simulink model "Control"  (R2022a)
settings: Solver=VariableStepAuto  StartTime=0.0  StopTime=10.0  RelTol=1e-3
libraries: slpidlib x6, robotcorelib x1
settings Model: LastModifiedBy=s389152

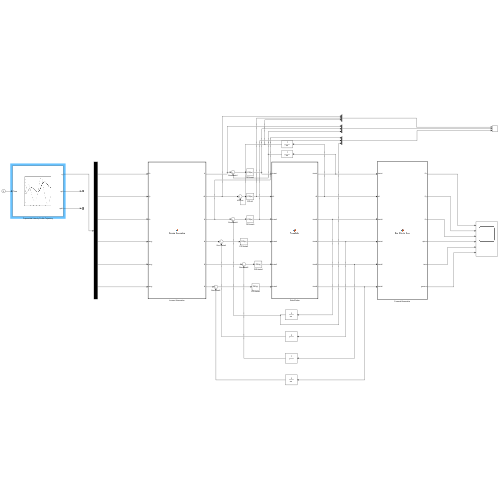
[thumbnail: Simulink's stored preview of the top-level diagram]
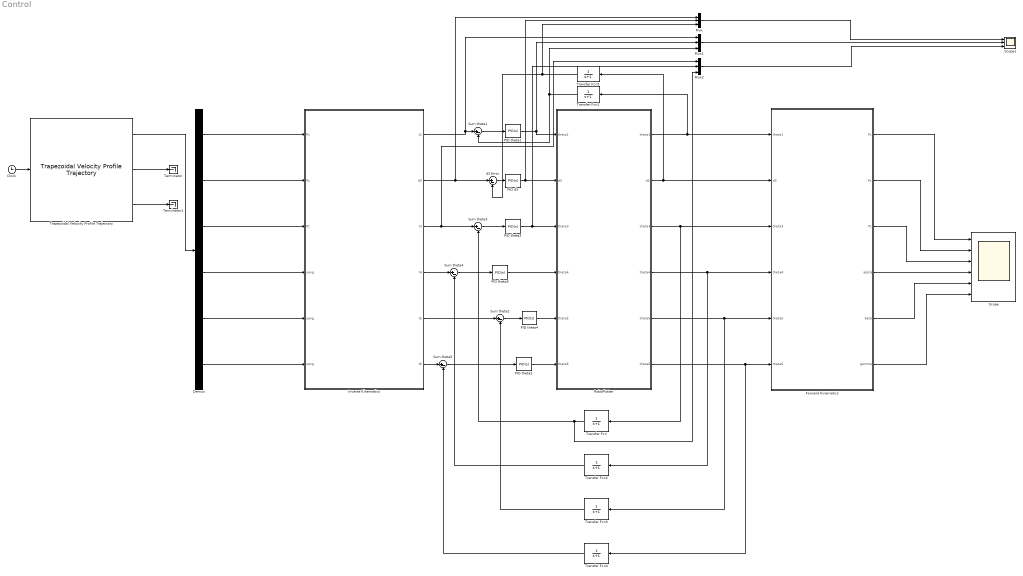
== system Control ==
  Clock : Clock
      settings: Decimation=5
  Demux : Demux  Outputs=6
  Forward Kinematics : MATLAB Function  TreatAsAtomicUnit=on
  Inverse Kinematics : MATLAB Function  TreatAsAtomicUnit=on
  Mux : Mux  Inputs=3
  Mux1 : Mux  Inputs=3
  Mux2 : Mux  Inputs=3
  PID d3 : slpidlib/PID Controller  Controller=PID  Form=Parallel  TimeDomain=Continuous-time  UseExternalTs=off  SampleTime=-1  IntegratorMethod=Forward Euler  FilterMethod=Forward Euler  ControllerParametersSource=internal  P=2  I=1.3  UseKiTs=off  D=.01  N=100  UseFilter=on  TunerSelectOption=Transfer Function Based (PID Tuner App)  InitialConditionSource=internal  InitialConditionForIntegrator=0  InitialConditionForFilter=0  DifferentiatorICPrevScaledInput=0  ExternalReset=none  TrackingMode=off  Kt=1  LimitOutput=off  SatLimitsSource=internal  UpperSaturationLimit=inf  LowerSaturationLimit=-inf  LinearizeAsGain=on  AntiWindupMode=none  Kb=1  POutMin=[]  POutMax=[]  IOutMin=[]  IOutMax=[]  DOutMin=[]  DOutMax=[]  NOutMin=[]  NOutMax=[]  SumOutMin=[]  SumOutMax=[]  SaturationOutMin=[]  SaturationOutMax=[]  PParamMin=[]  PParamMax=[]  IParamMin=[]  IParamMax=[]  DParamMin=[]  DParamMax=[]  NParamMin=[]  NParamMax=[]  KbParamMin=[]  KbParamMax=[]  KtParamMin=[]  KtParamMax=[]  KbOutMin=[]  KbOutMax=[]  KtOutMin=[]  KtOutMax=[]  IntegratorOutMin=[]  IntegratorOutMax=[]  FilterOutMin=[]  FilterOutMax=[]  SumI1OutMin=[]  SumI1OutMax=[]  SumI2OutMin=[]  SumI2OutMax=[]  SumI3OutMin=[]  SumI3OutMax=[]  SumI4OutMin=[]  SumI4OutMax=[]  SumDOutMin=[]  SumDOutMax=[]  DifferentiatorOutMin=[]  DifferentiatorOutMax=[]  FilterDiffOutCoefMin=[]  FilterDiffOutCoefMax=[]  ReciprocalOutMin=[]  ReciprocalOutMax=[]  SumDenOutMin=[]  SumDenOutMax=[]  SumNumOutMin=[]  SumNumOutMax=[]  DivideOutMin=[]  DivideOutMax=[]  UdiffTsProdOutMin=[]  UdiffTsProdOutMax=[]  NTsProdOutMin=[]  NTsProdOutMax=[]  UintegralTsProdOutMin=[]  UintegralTsProdOutMax=[]  UngainTsProdOutMin=[]  UngainTsProdOutMax=[]  IntegratorContinuousStateAttributes=''  IntegratorStateMustResolveToSignalObject=off  IntegratorRTWStateStorageClass=Auto  FilterContinuousStateAttributes=''  FilterStateMustResolveToSignalObject=off  FilterRTWStateStorageClass=Auto  ParallelPVariant=InternalParameters  IdealPVariant=Disabled  IVariant=InternalParameters  DVariant=InternalParameters  IntegratorVariant=Continuous  SatVariant=Disabled  AWVariant=Passthrough  PCopyVariant=Disabled  TRVariant=Disabled  FdbkBlocksVariant=Forward  IdealPFdbkVariant=Disabled  SatFdbkVariant=Disabled  DerivativeFilterVariant=ContFilter  NVariant=InternalParameters  NCopyVariant=Disabled  FilterICVariant=InternalICsFilter  IntegratorICVariant=InternalICs  ExternalResetVariant=Disabled  TRSumVariant=Passthrough  SumFdbkVariant=Disabled  SumVariant=Sum_PID  TsampFilterVariant=InternalTs  TsampNgainVariant=Passthrough  TsampIntegralVariant=Passthrough  ExternalSaturationOutDataTypeStr=Inherit: Same as second input  aMode=0
  PID theta1 : slpidlib/PID Controller  Controller=PID  Form=Parallel  TimeDomain=Continuous-time  UseExternalTs=off  SampleTime=-1  IntegratorMethod=Forward Euler  FilterMethod=Forward Euler  ControllerParametersSource=internal  P=1.3  I=1.3  UseKiTs=off  D=0.01  N=100  UseFilter=on  TunerSelectOption=Transfer Function Based (PID Tuner App)  InitialConditionSource=internal  InitialConditionForIntegrator=0  InitialConditionForFilter=0  DifferentiatorICPrevScaledInput=0  ExternalReset=none  TrackingMode=off  Kt=1  LimitOutput=off  SatLimitsSource=internal  UpperSaturationLimit=inf  LowerSaturationLimit=-inf  LinearizeAsGain=on  AntiWindupMode=none  Kb=1  POutMin=[]  POutMax=[]  IOutMin=[]  IOutMax=[]  DOutMin=[]  DOutMax=[]  NOutMin=[]  NOutMax=[]  SumOutMin=[]  SumOutMax=[]  SaturationOutMin=[]  SaturationOutMax=[]  PParamMin=[]  PParamMax=[]  IParamMin=[]  IParamMax=[]  DParamMin=[]  DParamMax=[]  NParamMin=[]  NParamMax=[]  KbParamMin=[]  KbParamMax=[]  KtParamMin=[]  KtParamMax=[]  KbOutMin=[]  KbOutMax=[]  KtOutMin=[]  KtOutMax=[]  IntegratorOutMin=[]  IntegratorOutMax=[]  FilterOutMin=[]  FilterOutMax=[]  SumI1OutMin=[]  SumI1OutMax=[]  SumI2OutMin=[]  SumI2OutMax=[]  SumI3OutMin=[]  SumI3OutMax=[]  SumI4OutMin=[]  SumI4OutMax=[]  SumDOutMin=[]  SumDOutMax=[]  DifferentiatorOutMin=[]  DifferentiatorOutMax=[]  FilterDiffOutCoefMin=[]  FilterDiffOutCoefMax=[]  ReciprocalOutMin=[]  ReciprocalOutMax=[]  SumDenOutMin=[]  SumDenOutMax=[]  SumNumOutMin=[]  SumNumOutMax=[]  DivideOutMin=[]  DivideOutMax=[]  UdiffTsProdOutMin=[]  UdiffTsProdOutMax=[]  NTsProdOutMin=[]  NTsProdOutMax=[]  UintegralTsProdOutMin=[]  UintegralTsProdOutMax=[]  UngainTsProdOutMin=[]  UngainTsProdOutMax=[]  IntegratorContinuousStateAttributes=''  IntegratorStateMustResolveToSignalObject=off  IntegratorRTWStateStorageClass=Auto  FilterContinuousStateAttributes=''  FilterStateMustResolveToSignalObject=off  FilterRTWStateStorageClass=Auto  ParallelPVariant=InternalParameters  IdealPVariant=Disabled  IVariant=InternalParameters  DVariant=InternalParameters  IntegratorVariant=Continuous  SatVariant=Disabled  AWVariant=Passthrough  PCopyVariant=Disabled  TRVariant=Disabled  FdbkBlocksVariant=Forward  IdealPFdbkVariant=Disabled  SatFdbkVariant=Disabled  DerivativeFilterVariant=ContFilter  NVariant=InternalParameters  NCopyVariant=Disabled  FilterICVariant=InternalICsFilter  IntegratorICVariant=InternalICs  ExternalResetVariant=Disabled  TRSumVariant=Passthrough  SumFdbkVariant=Disabled  SumVariant=Sum_PID  TsampFilterVariant=InternalTs  TsampNgainVariant=Passthrough  TsampIntegralVariant=Passthrough  ExternalSaturationOutDataTypeStr=Inherit: Same as second input  aMode=0
  PID theta2 : slpidlib/PID Controller  Controller=PID  Form=Parallel  TimeDomain=Continuous-time  UseExternalTs=off  SampleTime=-1  IntegratorMethod=Forward Euler  FilterMethod=Forward Euler  ControllerParametersSource=internal  P=1  I=1  UseKiTs=off  D=0  N=100  UseFilter=on  TunerSelectOption=Transfer Function Based (PID Tuner App)  InitialConditionSource=internal  InitialConditionForIntegrator=0  InitialConditionForFilter=0  DifferentiatorICPrevScaledInput=0  ExternalReset=none  TrackingMode=off  Kt=1  LimitOutput=off  SatLimitsSource=internal  UpperSaturationLimit=inf  LowerSaturationLimit=-inf  LinearizeAsGain=on  AntiWindupMode=none  Kb=1  POutMin=[]  POutMax=[]  IOutMin=[]  IOutMax=[]  DOutMin=[]  DOutMax=[]  NOutMin=[]  NOutMax=[]  SumOutMin=[]  SumOutMax=[]  SaturationOutMin=[]  SaturationOutMax=[]  PParamMin=[]  PParamMax=[]  IParamMin=[]  IParamMax=[]  DParamMin=[]  DParamMax=[]  NParamMin=[]  NParamMax=[]  KbParamMin=[]  KbParamMax=[]  KtParamMin=[]  KtParamMax=[]  KbOutMin=[]  KbOutMax=[]  KtOutMin=[]  KtOutMax=[]  IntegratorOutMin=[]  IntegratorOutMax=[]  FilterOutMin=[]  FilterOutMax=[]  SumI1OutMin=[]  SumI1OutMax=[]  SumI2OutMin=[]  SumI2OutMax=[]  SumI3OutMin=[]  SumI3OutMax=[]  SumI4OutMin=[]  SumI4OutMax=[]  SumDOutMin=[]  SumDOutMax=[]  DifferentiatorOutMin=[]  DifferentiatorOutMax=[]  FilterDiffOutCoefMin=[]  FilterDiffOutCoefMax=[]  ReciprocalOutMin=[]  ReciprocalOutMax=[]  SumDenOutMin=[]  SumDenOutMax=[]  SumNumOutMin=[]  SumNumOutMax=[]  DivideOutMin=[]  DivideOutMax=[]  UdiffTsProdOutMin=[]  UdiffTsProdOutMax=[]  NTsProdOutMin=[]  NTsProdOutMax=[]  UintegralTsProdOutMin=[]  UintegralTsProdOutMax=[]  UngainTsProdOutMin=[]  UngainTsProdOutMax=[]  IntegratorContinuousStateAttributes=''  IntegratorStateMustResolveToSignalObject=off  IntegratorRTWStateStorageClass=Auto  FilterContinuousStateAttributes=''  FilterStateMustResolveToSignalObject=off  FilterRTWStateStorageClass=Auto  ParallelPVariant=InternalParameters  IdealPVariant=Disabled  IVariant=InternalParameters  DVariant=InternalParameters  IntegratorVariant=Continuous  SatVariant=Disabled  AWVariant=Passthrough  PCopyVariant=Disabled  TRVariant=Disabled  FdbkBlocksVariant=Forward  IdealPFdbkVariant=Disabled  SatFdbkVariant=Disabled  DerivativeFilterVariant=ContFilter  NVariant=InternalParameters  NCopyVariant=Disabled  FilterICVariant=InternalICsFilter  IntegratorICVariant=InternalICs  ExternalResetVariant=Disabled  TRSumVariant=Passthrough  SumFdbkVariant=Disabled  SumVariant=Sum_PID  TsampFilterVariant=InternalTs  TsampNgainVariant=Passthrough  TsampIntegralVariant=Passthrough  ExternalSaturationOutDataTypeStr=Inherit: Same as second input  aMode=0
  PID theta3 : slpidlib/PID Controller  Controller=PID  Form=Parallel  TimeDomain=Continuous-time  UseExternalTs=off  SampleTime=-1  IntegratorMethod=Forward Euler  FilterMethod=Forward Euler  ControllerParametersSource=internal  P=1.3  I=1.3  UseKiTs=off  D=.01  N=100  UseFilter=on  TunerSelectOption=Transfer Function Based (PID Tuner App)  InitialConditionSource=internal  InitialConditionForIntegrator=0  InitialConditionForFilter=0  DifferentiatorICPrevScaledInput=0  ExternalReset=none  TrackingMode=off  Kt=1  LimitOutput=off  SatLimitsSource=internal  UpperSaturationLimit=inf  LowerSaturationLimit=-inf  LinearizeAsGain=on  AntiWindupMode=none  Kb=1  POutMin=[]  POutMax=[]  IOutMin=[]  IOutMax=[]  DOutMin=[]  DOutMax=[]  NOutMin=[]  NOutMax=[]  SumOutMin=[]  SumOutMax=[]  SaturationOutMin=[]  SaturationOutMax=[]  PParamMin=[]  PParamMax=[]  IParamMin=[]  IParamMax=[]  DParamMin=[]  DParamMax=[]  NParamMin=[]  NParamMax=[]  KbParamMin=[]  KbParamMax=[]  KtParamMin=[]  KtParamMax=[]  KbOutMin=[]  KbOutMax=[]  KtOutMin=[]  KtOutMax=[]  IntegratorOutMin=[]  IntegratorOutMax=[]  FilterOutMin=[]  FilterOutMax=[]  SumI1OutMin=[]  SumI1OutMax=[]  SumI2OutMin=[]  SumI2OutMax=[]  SumI3OutMin=[]  SumI3OutMax=[]  SumI4OutMin=[]  SumI4OutMax=[]  SumDOutMin=[]  SumDOutMax=[]  DifferentiatorOutMin=[]  DifferentiatorOutMax=[]  FilterDiffOutCoefMin=[]  FilterDiffOutCoefMax=[]  ReciprocalOutMin=[]  ReciprocalOutMax=[]  SumDenOutMin=[]  SumDenOutMax=[]  SumNumOutMin=[]  SumNumOutMax=[]  DivideOutMin=[]  DivideOutMax=[]  UdiffTsProdOutMin=[]  UdiffTsProdOutMax=[]  NTsProdOutMin=[]  NTsProdOutMax=[]  UintegralTsProdOutMin=[]  UintegralTsProdOutMax=[]  UngainTsProdOutMin=[]  UngainTsProdOutMax=[]  IntegratorContinuousStateAttributes=''  IntegratorStateMustResolveToSignalObject=off  IntegratorRTWStateStorageClass=Auto  FilterContinuousStateAttributes=''  FilterStateMustResolveToSignalObject=off  FilterRTWStateStorageClass=Auto  ParallelPVariant=InternalParameters  IdealPVariant=Disabled  IVariant=InternalParameters  DVariant=InternalParameters  IntegratorVariant=Continuous  SatVariant=Disabled  AWVariant=Passthrough  PCopyVariant=Disabled  TRVariant=Disabled  FdbkBlocksVariant=Forward  IdealPFdbkVariant=Disabled  SatFdbkVariant=Disabled  DerivativeFilterVariant=ContFilter  NVariant=InternalParameters  NCopyVariant=Disabled  FilterICVariant=InternalICsFilter  IntegratorICVariant=InternalICs  ExternalResetVariant=Disabled  TRSumVariant=Passthrough  SumFdbkVariant=Disabled  SumVariant=Sum_PID  TsampFilterVariant=InternalTs  TsampNgainVariant=Passthrough  TsampIntegralVariant=Passthrough  ExternalSaturationOutDataTypeStr=Inherit: Same as second input  aMode=0
  PID theta4 : slpidlib/PID Controller  Controller=PID  Form=Parallel  TimeDomain=Continuous-time  UseExternalTs=off  SampleTime=-1  IntegratorMethod=Forward Euler  FilterMethod=Forward Euler  ControllerParametersSource=internal  P=1  I=1  UseKiTs=off  D=0  N=100  UseFilter=on  TunerSelectOption=Transfer Function Based (PID Tuner App)  InitialConditionSource=internal  InitialConditionForIntegrator=0  InitialConditionForFilter=0  DifferentiatorICPrevScaledInput=0  ExternalReset=none  TrackingMode=off  Kt=1  LimitOutput=off  SatLimitsSource=internal  UpperSaturationLimit=inf  LowerSaturationLimit=-inf  LinearizeAsGain=on  AntiWindupMode=none  Kb=1  POutMin=[]  POutMax=[]  IOutMin=[]  IOutMax=[]  DOutMin=[]  DOutMax=[]  NOutMin=[]  NOutMax=[]  SumOutMin=[]  SumOutMax=[]  SaturationOutMin=[]  SaturationOutMax=[]  PParamMin=[]  PParamMax=[]  IParamMin=[]  IParamMax=[]  DParamMin=[]  DParamMax=[]  NParamMin=[]  NParamMax=[]  KbParamMin=[]  KbParamMax=[]  KtParamMin=[]  KtParamMax=[]  KbOutMin=[]  KbOutMax=[]  KtOutMin=[]  KtOutMax=[]  IntegratorOutMin=[]  IntegratorOutMax=[]  FilterOutMin=[]  FilterOutMax=[]  SumI1OutMin=[]  SumI1OutMax=[]  SumI2OutMin=[]  SumI2OutMax=[]  SumI3OutMin=[]  SumI3OutMax=[]  SumI4OutMin=[]  SumI4OutMax=[]  SumDOutMin=[]  SumDOutMax=[]  DifferentiatorOutMin=[]  DifferentiatorOutMax=[]  FilterDiffOutCoefMin=[]  FilterDiffOutCoefMax=[]  ReciprocalOutMin=[]  ReciprocalOutMax=[]  SumDenOutMin=[]  SumDenOutMax=[]  SumNumOutMin=[]  SumNumOutMax=[]  DivideOutMin=[]  DivideOutMax=[]  UdiffTsProdOutMin=[]  UdiffTsProdOutMax=[]  NTsProdOutMin=[]  NTsProdOutMax=[]  UintegralTsProdOutMin=[]  UintegralTsProdOutMax=[]  UngainTsProdOutMin=[]  UngainTsProdOutMax=[]  IntegratorContinuousStateAttributes=''  IntegratorStateMustResolveToSignalObject=off  IntegratorRTWStateStorageClass=Auto  FilterContinuousStateAttributes=''  FilterStateMustResolveToSignalObject=off  FilterRTWStateStorageClass=Auto  ParallelPVariant=InternalParameters  IdealPVariant=Disabled  IVariant=InternalParameters  DVariant=InternalParameters  IntegratorVariant=Continuous  SatVariant=Disabled  AWVariant=Passthrough  PCopyVariant=Disabled  TRVariant=Disabled  FdbkBlocksVariant=Forward  IdealPFdbkVariant=Disabled  SatFdbkVariant=Disabled  DerivativeFilterVariant=ContFilter  NVariant=InternalParameters  NCopyVariant=Disabled  FilterICVariant=InternalICsFilter  IntegratorICVariant=InternalICs  ExternalResetVariant=Disabled  TRSumVariant=Passthrough  SumFdbkVariant=Disabled  SumVariant=Sum_PID  TsampFilterVariant=InternalTs  TsampNgainVariant=Passthrough  TsampIntegralVariant=Passthrough  ExternalSaturationOutDataTypeStr=Inherit: Same as second input  aMode=0
  PID theta5 : slpidlib/PID Controller  Controller=PID  Form=Parallel  TimeDomain=Continuous-time  UseExternalTs=off  SampleTime=-1  IntegratorMethod=Forward Euler  FilterMethod=Forward Euler  ControllerParametersSource=internal  P=1  I=1  UseKiTs=off  D=0  N=100  UseFilter=on  TunerSelectOption=Transfer Function Based (PID Tuner App)  InitialConditionSource=internal  InitialConditionForIntegrator=0  InitialConditionForFilter=0  DifferentiatorICPrevScaledInput=0  ExternalReset=none  TrackingMode=off  Kt=1  LimitOutput=off  SatLimitsSource=internal  UpperSaturationLimit=inf  LowerSaturationLimit=-inf  LinearizeAsGain=on  AntiWindupMode=none  Kb=1  POutMin=[]  POutMax=[]  IOutMin=[]  IOutMax=[]  DOutMin=[]  DOutMax=[]  NOutMin=[]  NOutMax=[]  SumOutMin=[]  SumOutMax=[]  SaturationOutMin=[]  SaturationOutMax=[]  PParamMin=[]  PParamMax=[]  IParamMin=[]  IParamMax=[]  DParamMin=[]  DParamMax=[]  NParamMin=[]  NParamMax=[]  KbParamMin=[]  KbParamMax=[]  KtParamMin=[]  KtParamMax=[]  KbOutMin=[]  KbOutMax=[]  KtOutMin=[]  KtOutMax=[]  IntegratorOutMin=[]  IntegratorOutMax=[]  FilterOutMin=[]  FilterOutMax=[]  SumI1OutMin=[]  SumI1OutMax=[]  SumI2OutMin=[]  SumI2OutMax=[]  SumI3OutMin=[]  SumI3OutMax=[]  SumI4OutMin=[]  SumI4OutMax=[]  SumDOutMin=[]  SumDOutMax=[]  DifferentiatorOutMin=[]  DifferentiatorOutMax=[]  FilterDiffOutCoefMin=[]  FilterDiffOutCoefMax=[]  ReciprocalOutMin=[]  ReciprocalOutMax=[]  SumDenOutMin=[]  SumDenOutMax=[]  SumNumOutMin=[]  SumNumOutMax=[]  DivideOutMin=[]  DivideOutMax=[]  UdiffTsProdOutMin=[]  UdiffTsProdOutMax=[]  NTsProdOutMin=[]  NTsProdOutMax=[]  UintegralTsProdOutMin=[]  UintegralTsProdOutMax=[]  UngainTsProdOutMin=[]  UngainTsProdOutMax=[]  IntegratorContinuousStateAttributes=''  IntegratorStateMustResolveToSignalObject=off  IntegratorRTWStateStorageClass=Auto  FilterContinuousStateAttributes=''  FilterStateMustResolveToSignalObject=off  FilterRTWStateStorageClass=Auto  ParallelPVariant=InternalParameters  IdealPVariant=Disabled  IVariant=InternalParameters  DVariant=InternalParameters  IntegratorVariant=Continuous  SatVariant=Disabled  AWVariant=Passthrough  PCopyVariant=Disabled  TRVariant=Disabled  FdbkBlocksVariant=Forward  IdealPFdbkVariant=Disabled  SatFdbkVariant=Disabled  DerivativeFilterVariant=ContFilter  NVariant=InternalParameters  NCopyVariant=Disabled  FilterICVariant=InternalICsFilter  IntegratorICVariant=InternalICs  ExternalResetVariant=Disabled  TRSumVariant=Passthrough  SumFdbkVariant=Disabled  SumVariant=Sum_PID  TsampFilterVariant=InternalTs  TsampNgainVariant=Passthrough  TsampIntegralVariant=Passthrough  ExternalSaturationOutDataTypeStr=Inherit: Same as second input  aMode=0
  RoboPlotter : MATLAB Function  TreatAsAtomicUnit=on
  Scope : Scope  NumInputPorts=6
  Scope1 : Scope  NumInputPorts=3
  Sum theta{1..5} (5 alike) : Sum  Inputs=|+-
  Terminator : Terminator
  Terminator1 : Terminator
  Transfer Fcn{,1..5} (6 alike) : TransferFcn  Denominator="[1  1]"
  Trapezoidal Velocity Profile Trajectory : robotcorelib/Trapezoidal Velocity Profile Trajectory  WaypointSource=Internal  Waypoints="[ 2500, 2500; 400, 500; 0,0; 90,90; 0,0; 90,90;  ]"  NumParams=0  Parameter1=End Time  Parameter2=End Time  ParameterSource=Internal  PeakVelocity=[ 2; 2 ]  Acceleration=[ 1; 2 ]  EndTime=[ 1; 1 ]  AccelTime=[ 1; 2 ]  SimulateUsing=Interpreted execution
      settings: SourceProductBaseCode=RO,NV,RR,UV
  d3 Error : Sum  Inputs=|+-
  wires:
  Trapezoidal Velocity Profile Trajectory/3 -> Terminator1/1
  Trapezoidal Velocity Profile Trajectory/2 -> Terminator/1
  Trapezoidal Velocity Profile Trajectory/1 -> Demux/1
  Demux/1 -> Inverse Kinematics/1(Px)
  Demux/2 -> Inverse Kinematics/2(Py)
  Demux/3 -> Inverse Kinematics/3(Pz)
  Demux/4 -> Inverse Kinematics/4(xang)
  Demux/5 -> Inverse Kinematics/5(yang)
  Demux/6 -> Inverse Kinematics/6(zang)
  Sum theta1/1 -> PID theta1/1
  Inverse Kinematics/1(t1) -> Mux1/1, Sum theta1/1
  PID theta1/1 -> Mux1/2, RoboPlotter/1("theta1 ")
  Inverse Kinematics/2(d3) -> Mux/1, d3 Error/1
  PID d3/1 -> Mux/2, RoboPlotter/2("d3 ")
  RoboPlotter/2(d3) -> Transfer Fcn5/1, Forward Kinematics/2(d3)
  d3 Error/1 -> PID d3/1
  Inverse Kinematics/3(t3) -> Mux2/1, Sum theta3/1
  PID theta3/1 -> Mux2/2, RoboPlotter/3("theta3 ")
  RoboPlotter/3(theta3) -> Forward Kinematics/3(theta3), Transfer Fcn/1
  Sum theta3/1 -> PID theta3/1
  RoboPlotter/4(theta4) -> Transfer Fcn2/1, Forward Kinematics/4(theta4)
  RoboPlotter/5(theta5) -> Transfer Fcn3/1, Forward Kinematics/5(theta5)
  RoboPlotter/6(theta6) -> Transfer Fcn4/1, Forward Kinematics/6(theta6)
  Forward Kinematics/1(Px) -> Scope/1
  Forward Kinematics/2(Py) -> Scope/2
  RoboPlotter/1(theta1) -> Transfer Fcn1/1, Forward Kinematics/1(theta1)
  Clock/1 -> Trapezoidal Velocity Profile Trajectory/1
  Forward Kinematics/3(Pz) -> Scope/3
  Mux/1 -> Scope1/1
  Transfer Fcn/1 -> Sum theta3/2, Mux2/3
  Transfer Fcn1/1 -> Mux1/3, Sum theta1/2
  Mux1/1 -> Scope1/2
  Mux2/1 -> Scope1/3
  Inverse Kinematics/6(t6) -> Sum theta5/1
  Inverse Kinematics/4(t4) -> Sum theta4/1
  Inverse Kinematics/5(t5) -> Sum theta2/1
  Transfer Fcn2/1 -> Sum theta4/2
  Transfer Fcn3/1 -> Sum theta2/2
  Transfer Fcn4/1 -> Sum theta5/2
  Sum theta5/1 -> PID theta2/1
  Sum theta2/1 -> PID theta4/1
  Sum theta4/1 -> PID theta5/1
  PID theta5/1 -> RoboPlotter/4("theta4 ")
  PID theta4/1 -> RoboPlotter/5("theta5 ")
  PID theta2/1 -> RoboPlotter/6("theta6 ")
  Forward Kinematics/4(alpha) -> Scope/4
  Forward Kinematics/5(beta) -> Scope/5
  Forward Kinematics/6(gamma) -> Scope/6
  Transfer Fcn5/1 -> Mux/3, d3 Error/2

== matlab function Control/Forward Kinematics ==
  data: theta1 input; Px output; d3 input; theta3 input; theta4 input; theta5 input; theta6 input; Py output; Pz output; alpha output; beta output; gamma output
%Function to know the location of end effector 
function [Px, Py, Pz, alpha, beta, gamma]  = End_Effector_Loc(theta1, d3, theta3, theta4, theta5, theta6)
    mount_offset = [0;0;90;0;]; %offset between frame 7 and 6 (not included in DH parameter)
    TCP = mount_offset + [0;0;90;1;]; %deault value of TCP
    Trans = DH_param(d3, theta1, theta3, theta4, theta5, theta6); 
    T06 = Trans(:,21:24);
    %Frame6_0 = T06 * [0;0;0;1];
    eulerangle = (T06(1:3, 1:3));
    zyx = rotm2eul(eulerangle)*(180/pi);
    TCP_Global = T06 * TCP;
    Px = TCP_Global(1);
    Py = TCP_Global(2);
    Pz = TCP_Global(3);
    alpha = zyx(3);
    beta = zyx(2);
    gamma = zyx(1);
   end

%+++++++++++++++++++++++++++++++++++++++++++++++++++++++++++++++++++++++++++++++++++++++++++++++++++++



 %++++++++++++++++++++++++++++++++++++++++++++++++++++++++++++++++++++++++++++++++++++++

    

function  [trans]= DH_param (d3, theta1, theta3, theta4, theta5, theta6)

%Predifined values for the link offsets and link lengths
d1 = 400;
d5 = 1800;
a2 = 400;
a4 = 300;


%Function calls to calculate the transformation matrics for joint i wrt i-1
t01 = (Trans_Matrix(0, -90, d1, theta1));
t12 = (Trans_Matrix(a2, 0, d3, 0));
t23 = (Trans_Matrix(a4, 90, 0, (theta3+90)));
t34 = (Trans_Matrix(0, 90, d5, theta4));
t45 = (Trans_Matrix(0, -90, 0, theta5));
t56 = (Trans_Matrix(0, 90, 0, theta6));


%Calculation of overall transformation matrix from frame 0 to frame 7


t02 = (t01*t12);
t03 = (t01*t12*t23);
t04 = (t01*t12*t23*t34);
t05 = (t01*t12*t23*t34*t45);
t06 = (t01*t12*t23*t34*t45*t56);


trans = [t01, t02, t03, t04, t05, t06];
end

== matlab function Control/Inverse Kinematics ==
  data: Px input; t1 output; Py input; Pz input; xang input; yang input; zang input; d3 output; t3 output; t4 output; t5 output; t6 output
%Program to compute the inverse kinematics 

function [t1, d3, t3, t4, t5, t6]  = Inverse_kinematics(Px, Py, Pz, xang, yang, zang)
%Predifined values for the link offsets and link lengths
d1 = 400;
d5 = 1800;
a2 = 400;
a4 = 300;

%initialize set values to nan
set1 = [nan nan nan nan nan nan];
set2 = [nan nan nan nan nan nan];
set3 = [nan nan nan nan nan nan];
set4 = [nan nan nan nan nan nan];
set5 = [nan nan nan nan nan nan];
set6 = [nan nan nan nan nan nan];
set7 = [nan nan nan nan nan nan];
set8 = [nan nan nan nan nan nan];


%++++++++++++++++++++++++++++++++++++++++++++++++++++++++++++++++++++++++++++++++++++++

%TCP and wrist compensation

rotx = [1 0 0; 
        0 cosd(xang) -sind(xang); 
        0 sind(xang) cosd(xang);];
roty = [cosd(yang) 0 sind(yang);
        0 1 0; 
        -sind(yang) 0 cosd(yang);];
rotz = [cosd(zang) -sind(zang) 0; 
        sind(zang) cosd(zang) 0; 
        0 0 1;];
%----------------------------------------
Rot_overall = (rotz*roty*rotx);

pos = [Px; Py; Pz];

TCP =[0;0;90;];


newpos = pos - Rot_overall*TCP;
Px = newpos(1);
Py = newpos(2);
Pz = newpos(3);


%++++++++++++++++++++++++++++++++++++++++++++++++++++++++++++++++++++++++++++++++++++++
%Theta1
theta1 = -atan2d(Pz, Px);
if (theta1<-90 || theta1>90)
        theta1 = nan;
end
theta11 = theta1+180;
if (theta11<-90 || theta11>90)
    theta11 = nan;
end

%+_________________________________________________++++
%theta3

%To throw an error if theta3 would go complex
if (((Px/cosd(theta1)-a2 - a4)/d5)>1)
    error("SINGULARITY CONDITION");
end

theta3p = asind(((Px/cosd(theta1))-a2 - a4)/d5);
theta3 = 90-theta3p; %To measure wrt x3 and x4
if (theta3<-90 || theta3>90)
    theta3 = nan;
end

theta3a = -theta3;
if (theta3a<-90 || theta3a>90)
    theta3a = nan;
end

%++++++++++++++++++++++++++++++++++++++++++++++++++++++++++++++++++++++++++++++++++++++
%theta3 wrt theta1prime
theta33p = asind(((Px/cosd(theta11))-a2 - a4)/d5);
theta33 = 90-theta33p;
if (theta33<-90 || theta33>90)
    theta33 = nan;
end

theta33a = -theta33;
if (theta33a<-90 || theta33a>90)
    theta33a = nan;
end

%++++++++++++++++++++++++++++++++++++++++++++++++++++++++++++++++++++++++++++++++++++++
%d3
d3 = Py-d1-d5*sind(theta3);
if (d3<0 || d3>2500)
    d3 = nan;
end
d3a = Py-d1-d5*sind(theta3a);
if (d3a<0 || d3a>2500)
    d3a = nan;
end

%d3 wrt theta1prime
d33 = Py-d1-d5*sind(theta33);
if (d33<0 || d33>2500)
    d33 = nan;
end
d33a = Py-d1-d5*sind(theta33a);
if (d33a<0 || d33a>2500)
    d33a = nan;
end

%++++++++++++++++++++++++++++++++++++++++++++++++++++++++++++++++++++++++++++++++++++++
%Last three angles
if(isreal(theta1) && isreal(d3) && isreal(theta3))
    theta456a = IK_orientation(zang, yang, xang, theta1, d3, theta3);
end
if(isreal(theta1) && isreal(d3a) && isreal(theta3a))
    theta456aa = IK_orientation(zang, yang, xang, theta1, d3a, theta3a);
end
if(isreal(theta11) && isreal(d33) && isreal(theta33))
    theta456b = IK_orientation(zang, yang, xang, theta11, d33, theta33);
end
if(isreal(theta11) && isreal(d33a) && isreal(theta33a))
    theta456bb = IK_orientation(zang, yang, xang, theta11, d33a, theta33a);
end

%++++++++++++++++++++++++++++++++++++++++++++++++++++++++++++++++++++++++++++++++++++++
if(isreal(theta1) && isreal(d3) && isreal(theta3))
    joint_var_pos_S1 = [theta1 d3 theta3];
    joint_var_orient_S11 = [theta456a(1) theta456a(3) theta456a(5)];
    joint_var_orient_S12 = [theta456a(2) theta456a(4) theta456a(6)];

    set1 = [joint_var_pos_S1 joint_var_orient_S11];
    set2 = [joint_var_pos_S1 joint_var_orient_S12];
end

if(isreal(theta1) && isreal(d3a) && isreal(theta3a))
    joint_var_pos_S2 = [theta1 d3a theta3a];
    joint_var_orient_S21 = [theta456aa(1) theta456aa(3) theta456aa(5)];
    joint_var_orient_S22 = [theta456aa(2) theta456aa(4) theta456aa(6)];

    set3 = [joint_var_pos_S2 joint_var_orient_S21];
    set4 = [joint_var_pos_S2 joint_var_orient_S22];

end

if(isreal(theta11) && isreal(d33) && isreal(theta33))
    joint_var_pos_S3 = [theta11 d33 theta33];
    joint_var_orient_S31 = [theta456b(1) theta456b(3) theta456b(5)];
    joint_var_orient_S32 = [theta456b(2) theta456b(4) theta456b(6)];

    set5 = [joint_var_pos_S3 joint_var_orient_S31];
    set6 = [joint_var_pos_S3 joint_var_orient_S32];

end

if(isreal(theta11) && isreal(d33a) && isreal(theta33a))
    joint_var_pos_S4 = [theta11 d33a theta33a];
    joint_var_orient_S41 = [theta456bb(1) theta456bb(3) theta456bb(5)];
    joint_var_orient_S42 = [theta456bb(2) theta456bb(4) theta456bb(6)];

    set7 = [joint_var_pos_S4 joint_var_orient_S41];
    set8 = [joint_var_pos_S4 joint_var_orient_S42];

end
Jointvalues = [set1; set2; set3; set4; set5; set6; set7; set8;];




% %++++++++++++++++++++++++++++++++++++++++++++++++++++++++++++++++++++++++++++++++++++++
%To check if atleast one solution exists
flag = 0;
j = 1;
jointv = nan(8,6);
Workspace_cond = isnan(Jointvalues); %converts the joint value matrix to logical matrix

%Loop to check each row for non NAN values
for i = 1:8
    if any(Workspace_cond(i, :))
        flag = flag + 1;
    else
        jointv(j, :)  = Jointvalues(i,:);
        j = j+1;
        
    end
end

%flag will be 8 if all solutions has atleast one NAN any() returns 1 for
%such solutions
if flag == 8
   
    error("The point is out of work envelope No solution exist). Exiting...")

end

flag1 = 1;
Jointvalues =  jointv;

%return the set of values
t1 = Jointvalues(flag1, 1);
d3 = Jointvalues(flag1, 2);
t3 = Jointvalues(flag1, 3);
t4 = Jointvalues(flag1, 4);
t5 = Jointvalues(flag1, 5);
t6 = Jointvalues(flag1, 6);
%++++++++++++++++++++++++++++++++++++++++++++++++++++++++++++++++++++++++++++++++++++++


end

%++++++++++++++++++++++++++++++++++++++++++++++++++++++++++++++++++++++++++++++++++++++


function [theta567] = IK_orientation(zang, yang, xang, theta1, d3, theta3)

    %Program to compute the orientation part of the inverse kinematics
    
    
    rotx = [1 0 0; 
            0 cosd(xang) -sind(xang); 
            0 sind(xang) cosd(xang);];
    roty = [cosd(yang) 0 sind(yang);
            0 1 0; 
            -sind(yang) 0 cosd(yang);];
    rotz = [cosd(zang) -sind(zang) 0; 
            sind(zang) cosd(zang) 0; 
            0 0 1;];
    
    Rot_overall = (rotz*roty*rotx);
    trans = DH_param(d3, theta1, theta3, 0, 0, 0);
    rot_03  = trans(1:3, 9:11);
    rot_03Transpose = transpose(rot_03);
    Lrot_36 = (rot_03Transpose*Rot_overall);


    theta5 = (atan2d(sqrt((Lrot_36( 2,1))^2 + (Lrot_36(2,2))^2), -Lrot_36(2,3)));
    theta4 = (atan2d(-Lrot_36(3,3),  Lrot_36(1,3)));     
    theta6 = (atan2d(-Lrot_36(2,2),  Lrot_36(2,1)));

    theta5dash = -theta5;
    theta4dash = theta4 + 180;
    theta6dash = theta6 + 180;
    
    %To induce mechanical constrain to joint 5 
    
    if (theta5<-170 || theta5>170)
        theta5 = nan;
    end
    if (theta5dash<-170 || theta5dash>170)
        theta5dash = nan;
    end
    
    theta567 = [theta4 theta4dash theta5 theta5dash theta6 theta6dash];
    end
    
   %++++++++++++++++++++++++++++++++++++++++++++++++++++++++++++++++++++++++++++++++++++++

    

function  [trans]= DH_param (d3, theta1, theta3, theta4, theta5, theta6)

%Predifined values for the link offsets and link lengths
d1 = 400;
d5 = 1800;
a2 = 400;
a4 = 300;


%Function calls to calculate the transformation matrics for joint i wrt i-1
t01 = (Trans_Matrix(0, -90, d1, theta1));
t12 = (Trans_Matrix(a2, 0, d3, 0));
t23 = (Trans_Matrix(a4, 90, 0, (theta3+90)));
t34 = (Trans_Matrix(0, 90, d5, theta4));
t45 = (Trans_Matrix(0, -90, 0, theta5));
t56 = (Trans_Matrix(0, 90, 0, theta6));


%Calculation of overall transformation matrix from frame 0 to frame 7


t02 = (t01*t12);
t03 = (t01*t12*t23);
t04 = (t01*t12*t23*t34);
t05 = (t01*t12*t23*t34*t45);
t06 = (t01*t12*t23*t34*t45*t56);


trans = [t01, t02, t03, t04, t05, t06];
end

== matlab function Control/RoboPlotter ==
  data: theta1 input; theta1 output; d3 input; theta3 input; theta4 input; theta5 input; theta6 input; d3 output; theta3 output; theta4 output; theta5 output; theta6 output

function [theta1, d3, theta3, theta4, theta5, theta6] = Roboplotter(theta1, d3, theta3, theta4, theta5, theta6)

%Predifined values for the link offsets and link lengths
d1 = 400;
d5 = 1800;
a2 = 400;
a4 = 300;


%Function calls to calculate the transformation matrics for joint i wrt i-1
t01 = (Trans_Matrix(0, -90, d1, theta1));
t12 = (Trans_Matrix(a2, 0, d3, 0));
t23 = (Trans_Matrix(a4, 90, 0, (theta3+90)));
t34 = (Trans_Matrix(0, 90, d5, theta4));
t45 = (Trans_Matrix(0, -90, 0, theta5));
t56 = (Trans_Matrix(0, 90, 90, theta6));  %Mount offset incorporated


%Calculation of overall transformation matrix from frame 0 to frame 7


t02 = (t01*t12);
t03 = t02*t23;
t04 = t03*t34;
t05 = t04*t45;
t06 = (t05*t56);
p0 = [0;0;0;1];
p1 = t01(:, 4);
p2dash = p1 + [t01(1:3, 1:3)*[400;0;0];0];
p2 = t02(:, 4);
p3 = t03(:, 4);
p4 = t04(:, 4);
p5 = t05(:, 4);
p6 = t06(:, 4);
coordinates = [p0 p1 p2dash p2 p3 p4 p5 p6];
plot3(coordinates(1,:),coordinates(3,:),coordinates(2,:), 'r');
hold off

end
